simulink model "CruiseCtrl_StateFeedback"  (R2020a)
settings: Solver=ode45  StartTime=0.0  StopTime=40  MaxStep=0.01  RelTol=1e-3  EnableMultiTasking=on
values from neighbouring files (symbols this model uses):
  A = [[-1/tau 0];[1/m -rho*CD*Af*x2e/m]]    [CruiseCtrl_StateFeedback_Int_design.m]    (also in CruiseCtrl_StateFeedback_Int_design_EJ6.m = Aaug; Driveline_ctrl_design.m = [-ds/(Jf*i^2) ds/(Jf*i) -cs/(Jf*i); Driveline_ctrl_design_accion_int.m = [-ds/(Jf*i^2) ds/(Jf*i) -cs/(Jf*i); active_suspension_ctrl_design.m = [[0 1 0 0 0];[-(cw+cs)/mw -ds/mw cs/mw ds/mw -1/mw];[0 0 0 1)
  alpha = deg2rad(2)    [CruiseCtrl_StateFeedback_Int_design.m]    (also in CruiseCtrl_StateFeedback_Int_design_EJ6.m)
  B1 = [B H]    [CruiseCtrl_StateFeedback_Int_design.m]    (also in CruiseCtrl_StateFeedback_Int_design_EJ6.m = [Baug Haug]; Driveline_ctrl_design.m; Driveline_ctrl_design_accion_int.m; active_suspension_ctrl_design.m)
  C1 = eye(2)    [CruiseCtrl_StateFeedback_Int_design.m]    (also in CruiseCtrl_StateFeedback_Int_design_EJ6.m = eye(3); active_suspension_ctrl_design.m = eye(5))
  D1 = zeros(2)    [CruiseCtrl_StateFeedback_Int_design.m]    (also in CruiseCtrl_StateFeedback_Int_design_EJ6.m = zeros(3); active_suspension_ctrl_design.m = zeros(5,2))
  g = 9.82    [CruiseCtrl_StateFeedback_Int_design.m]    (also in CruiseCtrl_StateFeedback_Int_design_EJ6.m)
  K = acker(A,B,polos)    [CruiseCtrl_StateFeedback_Int_design.m]    (also in CruiseCtrl_StateFeedback_Int_design_EJ6.m = Kaug(1, 1:2); Driveline_ctrl_design.m; active_suspension_ctrl_design.m = lqr(A,B,Qx,Qu))
  kr = -1 / X    [CruiseCtrl_StateFeedback_Int_design.m]    (also in CruiseCtrl_StateFeedback_Int_design_EJ6.m; Driveline_ctrl_design.m; active_suspension_ctrl_design.m)
  ue = rw*x1e/k/r    (= 0.201)    [CruiseCtrl_StateFeedback_Int_design.m]    (also in CruiseCtrl_StateFeedback_Int_design_EJ6.m = 0.385125)
  x1e = 0.5*rho*CD*Af*x2e^2+m*g*f    (= 3216)    [CruiseCtrl_StateFeedback_Int_design.m]    (also in CruiseCtrl_StateFeedback_Int_design_EJ6.m = 6162)
  x2e = 15    [CruiseCtrl_StateFeedback_Int_design.m]    (also in CruiseCtrl_StateFeedback_Int_design_EJ6.m)
settings Model: Creator=JonasMac  LastModifiedBy=Adriana
settings DataIOCC: LimitDataPoints=on  SaveFormat=Array  ReturnWorkspaceOutputs=off
settings OptimizationCC: LifeSpan=inf
settings DebuggingCC: UnderspecifiedInitializationDetection=Classic  MergeDetectMultiDrivingBlocksExec=none  SolverPrmCheckMsg=warning  SFUnexpectedBacktrackingDiag=warning  SFNoUnconditionalDefaultTransitionDiag=warning  SFExecutionAtInitializationDiag=none  ArithmeticOperatorsInVariantConditions=warning
settings HardwareCC: ProdBitPerPointer=32  ProdBitPerSizeT=32  ProdBitPerPtrDiffT=32  ProdLargestAtomicFloat=None  ProdIntDivRoundTo=Undefined  ProdEndianess=Unspecified  ProdWordSize=32  ProdHWDeviceType=32-bit Generic
settings ModelReferenceCC: PropagateSignalLabelsOutOfModel=off
settings SFSimCC: SimUseLocalCustomCode=off  CustomCodeUndefinedFunction=UseInterfaceOnly
settings RTWCC: RTWUseLocalCustomCode=off
settings CodeAppCC: StateflowObjectComments=on
settings GRTTargetCC: TargetLangStandard=C89/C90 (ANSI)
settings ConfigComp: CovMetricSettings=dw  CovHtmlReporting=on  CovSaveCumulativeToWorkspaceVar=on  CovSaveSingleToWorkspaceVar=on  CovExternalEMLEnable=off

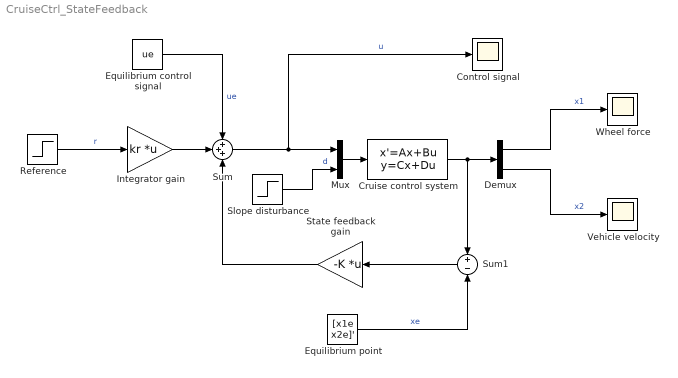
== system CruiseCtrl_StateFeedback ==
  Control signal : Scope
  Cruise control system : StateSpace  A=A  B=B1  C=C1  D=D1
  Demux : Demux  Outputs=2
  Equilibrium control signal : Constant  Value=ue
  "Equilibrium point " : Constant  Value=[x1e x2e]'
  Integrator gain : Gain  Gain=kr  Multiplication=Matrix(K*u)
  Mux : Mux  Inputs=2
  Reference : Step  After=5  SampleTime=0
  Slope disturbance : Step  Time=20  After=g*sin(alpha)  SampleTime=0
  State feedback gain : Gain  Gain=-K  Multiplication=Matrix(K*u)
  Sum : Sum  Inputs=+++
  Sum1 : Sum  Inputs=+-
  Vehicle velocity : Scope
  Wheel force : Scope
  wires:
  Demux/1 -> Wheel force/1  "x1"
  Demux/2 -> Vehicle velocity/1  "x2"
  Sum/1 -> Mux/1, Control signal/1  "u"
  Slope disturbance/1 -> Mux/2  "d"
  Integrator gain/1 -> Sum/2
  Equilibrium control signal/1 -> Sum/1  "ue"
  Cruise control system/1 -> Demux/1, Sum1/1
  Mux/1 -> Cruise control system/1
  State feedback gain/1 -> Sum/3
  Sum1/1 -> State feedback gain/1
  "Equilibrium point "/1 -> Sum1/2  "xe"
  Reference/1 -> Integrator gain/1  "r"
